simulink model "sf_gfexport"  (Simulink 6.0)
settings: Solver=ode45  StartTime=0.0  StopTime=inf  RelTol=1e-3
libraries: simulink x1
settings Model: CovMetricSettings=dcmtr  Creator=The MathWorks Inc.  LastModifiedBy=batserve  ExtModeAutoUpdateStatusClock=off
settings OptimizationCC: BooleanDataType=off
settings DebuggingCC: CheckExecutionContextPreStartOutputMsg=on  CheckExecutionContextRuntimeOutputMsg=on  SolverPrmCheckMsg=none
settings HardwareCC: TargetUnknown=on

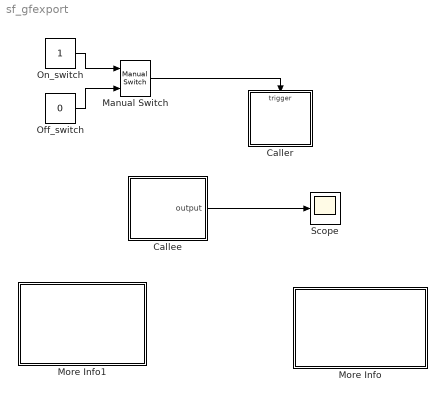
== system sf_gfexport ==
  Callee : Stateflow chart  PropExecContextAcrossSSBoundary=on
  Caller : Stateflow chart  TreatAsAtomicUnit=on  PropExecContextAcrossSSBoundary=on
  Manual Switch : simulink/Signal Routing/Manual Switch  sw=0  action=0
  More Info : Subsystem  PropExecContextAcrossSSBoundary=on
      mask Display: disp('Double click\nhere for\ninformation on\nthis demonstration')
  More Info1 : Subsystem  PropExecContextAcrossSSBoundary=on
      settings: OpenFcn=simcad(bdroot);
      mask Display: disp('Double click\nhere for\nSimulink\Stateflow\n Help')
  Off_switch : Constant  Value=0
  On_switch : Constant
  Scope : Scope
      settings: TimeRange=10  YMin=-1  YMax=1.3
  wires:
  On_switch/1 -> Manual Switch/1
  Off_switch/1 -> Manual Switch/2
  Manual Switch/1 -> Caller/Trigger
  Callee/1(output) -> Scope/1

== system sf_gfexport/More Info ==
  note: Graphical Function Demonstration
  note: This demonstration illustrates how graphical functions can be exported and used as a means for
      | accessing data. The output shown in the scope block, is equal to 1 when the manual switch is in the
      | On_switch state, or 0 when the switch is in the Off_switch state.
      |
      | The Caller chart is triggered by the Manual Switch. Graphical functions which are defined in the Callee
      | chart, are then called by the Caller chart. In the Callee chart, the output is set to 0 in state A and set to
      | 1 in state B. The graphical functions which are called by the Caller chart, first check if state A is active
      | and then send and transition even signal to the appropriate state. This method allows you to create
      | flexible models which contain different triggering events that define the final output.

== system sf_gfexport/More Info1 ==

== stateflow chart Caller ==
  (junction 4) -> (junction 3) : [is_A_active()]
      | {send_event_to_A();}
  (junction 4) -> (junction 3) : {send_event_to_B();}
  (default) -> (junction 4)
  events: E input EITHER_EDGE_EVENT

== stateflow chart Callee ==
  state A
    entry: output = 0;
  state B
    entry: output = 1;
  state activity = is_A_active() [function]
    (default) -> (junction 16) : {activity = in(A);}
  state send_event_to_A() [function]
    (default) -> (junction 17) : {send(SWITCH,A);}
  state send_event_to_B() [function]
    (default) -> (junction 18) : {send(SWITCH,B);}
  (default) -> A
  B -> A : SWITCH
  A -> B : SWITCH
  data: activity function_output double; output output double
  events: SWITCH local EITHER_EDGE_EVENT
